simulink model "Modele_LQR_6DOF_EXPERIMENTATION"  (R2024b)
settings: Solver=VariableStepAuto  StartTime=0.0  StopTime=30  FixedStep=0.0001  RelTol=1e-3
values from neighbouring files (symbols this model uses):
  A_num = [0 0 0 0 0 0 0 0 0 0 0 0 ... (144 elements, 12x12)]    [Matrice_A_lineaire.mat]    (also in calcul_matrice_A_lineaire.m = double(A_num); resultats_stabilite.mat; testFinale.m = A_fcn(0, 0, 0, val_rll, val_ptc, val_yw, val_u, val_v, val_w; test_calcalV2.m = double(A_num))
  B = df_dcontrol    [Generate_PyMatrix.m]    (also in Parameters.m = -234.459; instabiliter_graphique.m = out.B_s.signals.values)
  Fx1 = -0.7071*force    (= -0.7071)    [Parameters.m]
  Fx2 = -0.7071*force    (= -0.7071)    [Parameters.m]
  Fx3 = 0    [Parameters.m]
  Fx4 = 0    [Parameters.m]
  Fx5 = 0    [Parameters.m]
  Fx6 = 0    [Parameters.m]
  Fx7 = 0.7071*force    (= 0.7071)    [Parameters.m]
  Fx8 = 0.7071*force    (= 0.7071)    [Parameters.m]
  Fy1 = 0.7071*force    (= 0.7071)    [Parameters.m]
  Fy2 = -0.7071*force    (= -0.7071)    [Parameters.m]
  Fy3 = 0    [Parameters.m]
  Fy4 = 0    [Parameters.m]
  Fy5 = 0    [Parameters.m]
  Fy6 = 0    [Parameters.m]
  Fy7 = 0.7071*force    (= 0.7071)    [Parameters.m]
  Fy8 = -0.7071*force    (= -0.7071)    [Parameters.m]
  Fz1 = 0    [Parameters.m]
  Fz2 = 0    [Parameters.m]
  Fz3 = -1*force    (= -1)    [Parameters.m]
  Fz4 = -1*force    (= -1)    [Parameters.m]
  Fz5 = -1*force    (= -1)    [Parameters.m]
  Fz6 = -1*force    (= -1)    [Parameters.m]
  Fz7 = 0    [Parameters.m]
  Fz8 = 0    [Parameters.m]
  I_x = 0.578    [Parameters.m]
  I_y = 0.645    [Parameters.m]
  I_z = 0.9366    [Parameters.m]
  lx1 = 0.2987    [Parameters.m]
  lx2 = 0.2987    [Parameters.m]
  lx3 = -0.1073    [Parameters.m]
  lx4 = -0.1073    [Parameters.m]
  lx5 = 0.1073    [Parameters.m]
  lx6 = 0.1073    [Parameters.m]
  lx7 = -0.2987    [Parameters.m]
  lx8 = -0.2987    [Parameters.m]
  ly1 = 0.2130    (= 0.213)    [Parameters.m]
  ly2 = -0.2130    (= -0.213)    [Parameters.m]
  ly3 = 0.2725    [Parameters.m]
  ly4 = -0.2725    [Parameters.m]
  ly5 = 0.2725    [Parameters.m]
  ly6 = -0.2725    [Parameters.m]
  ly7 = 0.2130    (= 0.213)    [Parameters.m]
  ly8 = -0.2130    (= -0.213)    [Parameters.m]
  lz1 = 0    [Parameters.m]
  lz2 = 0    [Parameters.m]
  lz3 = 0    [Parameters.m]
  lz4 = 0    [Parameters.m]
  lz5 = 0    [Parameters.m]
  lz6 = 0    [Parameters.m]
  lz7 = 0    [Parameters.m]
  lz8 = 0    [Parameters.m]
  m = 0.427    [Calcul_Inertie_Nouveau.m]    (also in Parameters.m = 23.9)
  Q_envoyer = Q_final(:,:,1)    [Parameters.m]
  W = mass*gravity    (= 234.459)    [Generate_PyMatrix.m]    (also in Parameters.m; calcul_damping.m)
  x_rb = 0    [Parameters.m]
  x_rg = 0    [Parameters.m]
  y_rb = 0    [Parameters.m]
  y_rg = 0    [Parameters.m]
  z_rb = 0    [Parameters.m]
  z_rg = 0    [Parameters.m]
undefined symbols (not defined in the file or in its folder): sigbuilder_block
libraries: simulink x12, sharedtransform x1, dspinverses x1, SignalEditorBlockLib x1
(part 2 of 3)

== matlab function Modele_LQR_6DOF_EXPERIMENTATION/ROV model/ROV model/Kinetics1 ==
  data: u input size=1; u_dot output; v input size=1; w input size=1; p input size=1; q input size=1; r input size=1; phi input; theta input; psi input; tau input; v_dot output; w_dot output; p_dot output; q_dot output; r_dot output; u_dot_temp input; v_dot_temp input; w_dot_temp input; p_dot_temp input; q_dot_temp input; r_dot_temp input; disturbance input; EstimatedParams input; B parameter; Fx1 input; Fx2 input; Fx3 input; Fx4 input; Fx5 input; Fx6 input; Fx7 input; Fx8 input; Fy1 input; Fy2 input; Fy3 input; Fy4 input; Fy5 input; Fy6 input; Fy7 input; Fy8 input; Fz1 input; Fz2 input; Fz3 input; Fz4 input; Fz5 input; Fz6 input; Fz7 input; Fz8 input; I_x input; I_y input; I_z input; lx1 input; lx2 input; lx3 input; lx4 input; lx5 input; lx6 input; lx7 input; lx8 input; ly1 input; ly2 input; ly3 input; ly4 input; ly5 input; ly6 input; ly7 input; ly8 input; lz1 input; lz2 input; lz3 input; lz4 input; lz5 input; lz6 input; lz7 input; lz8 input; m parameter; W parameter; x_rb parameter; x_rg parameter; y_rb parameter; y_rg parameter; z_rb parameter; z_rg parameter; data output; ForceTotal output
function [u_dot, v_dot, w_dot, p_dot, q_dot, r_dot, data, ForceTotal] = Kinetics1( ...
    u, v, w, p, q, r, phi, theta, psi, tau, ...
    u_dot_temp, v_dot_temp, w_dot_temp, p_dot_temp, q_dot_temp, r_dot_temp, ...
    disturbance, EstimatedParams, B, ...
    Fx1, Fx2, Fx3, Fx4, Fx5, Fx6, Fx7, Fx8, ...
    Fy1, Fy2, Fy3, Fy4, Fy5, Fy6, Fy7, Fy8, ...
    Fz1, Fz2, Fz3, Fz4, Fz5, Fz6, Fz7, Fz8, ...
    I_x, I_y, I_z, ...
    lx1, lx2, lx3, lx4, lx5, lx6, lx7, lx8, ...
    ly1, ly2, ly3, ly4, ly5, ly6, ly7, ly8, ...
    lz1, lz2, lz3, lz4, lz5, lz6, lz7, lz8, ...
    m, W, x_rb, x_rg, y_rb, y_rg, z_rb, z_rg)
% ROV 6-DOF Kinetics — Newton-Euler equations (Fossen, p.58)
%
% INPUTS:
%   [u,v,w]         — linear velocities, body frame (m/s)
%   [p,q,r]         — angular velocities, body frame (rad/s)
%   [phi,theta,psi] — Euler angles (rad)
%   tau             — thruster forces (8x1, N)
%   [*_dot_temp]    — previous-step accelerations (breaks angular/linear circularity)
%   disturbance     — current disturbances [uc,vc,wc,pc,qc,rc]
%   EstimatedParams — hydrodynamic coefficients (18x1)
%   B, W            — buoyancy and weight (N)
%   Fx/Fy/Fzi       — unit force direction cosines for thruster i
%   I_x/y/z         — moments of inertia (kg.m²)
%   lx/ly/lzi       — moment arms for thruster i (m)
%   m               — mass (kg)
%   x/y/z_rb/rg     — buoyancy / gravity centre offsets (m)

% ── Constants (hardcoded — remove overrides to use argument values) ───
m    = 23.9;
B    = W;       % neutral buoyancy: (B-W)=0, all gX/gY/gZ terms vanish

x_rg = 0; y_rg = 0; z_rg = 0;
x_rb = 0; y_rb = 0; z_rb = 0;

% ── Previous-step accelerations (avoid circular dependency) ───────────
% p_dot/q_dot/r_dot depend on u_dot/v_dot/w_dot of the same step,
% so we use the delayed integrator feedback values instead.
ud = u_dot_temp;
vd = v_dot_temp;
wd = w_dot_temp;

% ── Hydrodynamic coefficients ─────────────────────────────────────────
X_u  = EstimatedParams(1);   Y_v  = EstimatedParams(2);
Z_w  = EstimatedParams(3);   K_p  = EstimatedParams(4);
M_q  = EstimatedParams(5);   N_r  = EstimatedParams(6);
X_uu = EstimatedParams(7);   Y_vv = EstimatedParams(8);
Z_ww = EstimatedParams(9);   K_pp = EstimatedParams(10);
M_qq = EstimatedParams(11);  N_rr = EstimatedParams(12);
X_ud = EstimatedParams(13);  Y_vd = EstimatedParams(14);
Z_wd = EstimatedParams(15);  K_pd = EstimatedParams(16);
M_qd = EstimatedParams(17);  N_rd = EstimatedParams(18);

% ── Current disturbances ──────────────────────────────────────────────
u_c = disturbance(1);  v_c = disturbance(2);  w_c = disturbance(3);
p_c = disturbance(4);  q_c = disturbance(5);  r_c = disturbance(6);

% ── Relative velocities ───────────────────────────────────────────────
ur = u - u_c;  vr = v - v_c;  wr = w - w_c;
pr = p - p_c;  qr = q - q_c;  rr = r - r_c;

% ── Trig ──────────────────────────────────────────────────────────────
sphi = sin(phi);  cphi = cos(phi);
sth  = sin(theta); cth = cos(theta);

% ── Thruster arrays ───────────────────────────────────────────────────
Fx = [Fx1 Fx2 Fx3 Fx4 Fx5 Fx6 Fx7 Fx8];
Fy = [Fy1 Fy2 Fy3 Fy4 Fy5 Fy6 Fy7 Fy8];
Fz = [Fz1 Fz2 Fz3 Fz4 Fz5 Fz6 Fz7 Fz8];
lx = [lx1 lx2 lx3 lx4 lx5 lx6 lx7 lx8];
ly = [ly1 ly2 ly3 ly4 ly5 ly6 ly7 ly8];
lz = [lz1 lz2 lz3 lz4 lz5 lz6 lz7 lz8];
f  = tau(1:8)';

% ── Generalised thruster forces and moments ───────────────────────────
tauX = sum(Fx .* f);
tauY = sum(Fy .* f);
tauZ = sum(Fz .* f);
tauK = sum((Fy.*lz - Fz.*ly) .* f);
tauM = sum((Fx.*lz - Fz.*lx) .* f);
tauN = sum((Fx.*ly - Fy.*lx) .* f);

% ══════════════════════════════════════════════════════════════════════
% Equations of motion — each variable isolated on the LHS
% All terms reproduced faithfully from original; only layout changed.
% ══════════════════════════════════════════════════════════════════════

% ── u_dot (surge) ────────────────────────────────────────────────────
u_dot = -(  (X_u + X_uu*abs(ur))*ur ...           % damping
          + tauX ...                               % thrusters
          + (q*w_c - r*v_c)*(X_ud - m) ...        % current-rate Coriolis
          + (Z_wd*wr + m*x_rg*qr)*qr ...
          - (Y_vd*vr - m*x_rg*rr)*rr ...
          + sth*(B - W) ...                        % restoring (=0 if B=W)
          - (m*y_rg*qr + m*z_rg*rr)*pr ...
          - m*qr*wr + m*rr*vr ...
          - m*q_dot_temp*z_rg + m*r_dot_temp*y_rg ...
         ) / (X_ud - m);

% ── v_dot (sway) ─────────────────────────────────────────────────────
v_dot = -(  (Y_v + Y_vv*abs(vr))*vr ...
          + tauY ...
          - (p*w_c - r*u_c)*(Y_vd - m) ...
          + (X_ud*ur + m*y_rg*rr)*rr ...
          - (Z_wd*wr - m*y_rg*pr)*pr ...
          - (m*x_rg*pr + m*z_rg*rr)*qr ...
          + m*pr*wr - m*rr*ur ...
          - cth*sphi*(B - W) ...
          + m*p_dot_temp*z_rg - m*r_dot_temp*x_rg ...
         ) / (Y_vd - m);

% ── w_dot (heave) ────────────────────────────────────────────────────
w_dot = -(  (Z_w + Z_ww*abs(wr))*wr ...
          + tauZ ...
          + (p*v_c - q*u_c)*(Z_wd - m) ...
          + (Y_vd*vr + m*z_rg*pr)*pr ...
          - (X_ud*ur - m*z_rg*qr)*qr ...
          - (m*x_rg*pr + m*y_rg*qr)*rr ...
          - m*pr*vr + m*qr*ur ...
          - cphi*cth*(B - W) ...
          - m*p_dot_temp*y_rg + m*q_dot_temp*x_rg ...
         ) / (Z_wd - m);

% ── p_dot (roll) ─────────────────────────────────────────────────────
p_dot = -(  (K_p + K_pp*abs(pr))*pr ...
          + tauK ...
          + (Y_vd*vr + m*z_rg*pr)*wr ...
          - (Z_wd*wr - m*y_rg*pr)*vr ...
          - cth*(W*y_rg*cphi - W*z_rg*sphi - B*y_rb*cphi + B*z_rb*sphi) ...
          - (m*y_rg*qr + m*z_rg*rr)*ur ...
          - (I_y*qr - M_qd*qr)*rr ...
          + (I_z*rr - N_rd*rr)*qr ...
          + m*y_rg*(wd + p*v_c - q*u_c) ...
          - m*z_rg*(vd - p*w_c + r*u_c) ...
         ) / (I_x - K_pd);

% ── q_dot (pitch) ────────────────────────────────────────────────────
q_dot = (   (M_q + M_qq*abs(qr))*qr ...
          + tauM ...
          - (Z_wd*wr + m*x_rg*qr)*ur ...
          + (X_ud*ur - m*z_rg*qr)*wr ...
          - (I_x*pr - K_pd*pr)*rr ...
          + (m*x_rg*pr + m*z_rg*rr)*vr ...
          + (I_z*rr - N_rd*rr)*pr ...
          + B*z_rb*sth - W*z_rg*sth ...
          + m*x_rg*(wd + p*v_c - q*u_c) ...
          - m*z_rg*(ud + q*w_c - r*v_c) ...
          + B*x_rb*cphi*cth - W*x_rg*cphi*cth ...
        ) / (I_y - M_qd);

% ── r_dot (yaw) ──────────────────────────────────────────────────────
r_dot = -(  (N_r + N_rr*abs(rr))*rr ...
          + tauN ...
          + (X_ud*ur + m*y_rg*rr)*vr ...
          - (Y_vd*vr - m*x_rg*rr)*ur ...
          - (I_x*pr - K_pd*pr)*qr ...
          + (I_y*qr - M_qd*qr)*pr ...
          - (m*x_rg*pr + m*y_rg*qr)*wr ...
          + B*y_rb*sth - W*y_rg*sth ...
          + m*x_rg*(vd - p*w_c + r*u_c) ...
          - m*y_rg*(ud + q*w_c - r*v_c) ...
          + B*x_rb*cth*sphi - W*x_rg*cth*sphi ...
         ) / (I_z - N_rd);

data = [ ...
u v w p q r ...
ur vr wr pr qr rr ...
u_dot v_dot w_dot p_dot q_dot r_dot];
ForceTotal = [tauX tauY tauZ tauK tauM tauN];
end

== matlab function Modele_LQR_6DOF_EXPERIMENTATION/Controller/MATLAB Function ==
  settings: updateMethod=DISCRETE
  data: R output; Q output; A output; B output; state input; Q_files input; A_lineraire input

function [R,Q,A,B]= ABmatrix(state, Q_files, A_lineraire)
tic
    
    roll_ = state(4);
    pitch_ = state(5);
    yaw_ = state(6);
    u = state(7); %
    v = state(8); %
    w = state(9); %
    p = state(10);
    q = state(11);
    r = state(12);
    thrust = 10;
    importance = 0;

    % Q = Q_files;
    Q = diag([Q_files(1,1)+200 Q_files(2,2)+200 Q_files(3,3)+200 Q_files(4,4) Q_files(5,5) Q_files(6,6) Q_files(7,7) Q_files(8,8) Q_files(9,9) Q_files(10,10) Q_files(11,11) Q_files(12,12)]);
    % Q = diag([80, 80, 80, 40, 40, 40, 20, 20, 20, 20, 20, 20]); % test répétition
    % Q = diag([4, 4, 4, 2, 2, 2, 1, 1, 1, 1, 1, 1]); % test ancien
    % R = diag([thrust, thrust, thrust-importance, thrust-importance, thrust-importance, thrust-importance, thrust, thrust]); 
    R = thrust*eye(8);

    radius = 0.26;
    
 % A = A_lineraire;

 % utiliser
%     A = [[0, 0, 0,   v*(sin(roll_)*sin(yaw_) + cos(roll_)*cos(yaw_)*sin(pitch_)) + w*(cos(roll_)*sin(yaw_) - cos(yaw_)*sin(pitch_)*sin(roll_)), w*cos(pitch_)*cos(roll_)*cos(yaw_) - u*cos(yaw_)*sin(pitch_) + v*cos(pitch_)*cos(yaw_)*sin(roll_), w*(cos(yaw_)*sin(roll_) - cos(roll_)*sin(pitch_)*sin(yaw_)) - v*(cos(roll_)*cos(yaw_) + sin(pitch_)*sin(roll_)*sin(yaw_)) - u*cos(pitch_)*sin(yaw_), cos(pitch_)*cos(yaw_), cos(yaw_)*sin(pitch_)*sin(roll_) - cos(roll_)*sin(yaw_), sin(roll_)*sin(yaw_) + cos(roll_)*cos(yaw_)*sin(pitch_),             0,                      0,                      0]
% [0, 0, 0, - v*(cos(yaw_)*sin(roll_) - cos(roll_)*sin(pitch_)*sin(yaw_)) - w*(cos(roll_)*cos(yaw_) + sin(pitch_)*sin(roll_)*sin(yaw_)), w*cos(pitch_)*cos(roll_)*sin(yaw_) - u*sin(pitch_)*sin(yaw_) + v*cos(pitch_)*sin(roll_)*sin(yaw_), w*(sin(roll_)*sin(yaw_) + cos(roll_)*cos(yaw_)*sin(pitch_)) - v*(cos(roll_)*sin(yaw_) - cos(yaw_)*sin(pitch_)*sin(roll_)) + u*cos(pitch_)*cos(yaw_), cos(pitch_)*sin(yaw_), cos(roll_)*cos(yaw_) + sin(pitch_)*sin(roll_)*sin(yaw_), cos(roll_)*sin(pitch_)*sin(yaw_) - cos(yaw_)*sin(roll_),             0,                      0,                      0]
% [0, 0, 0,                                                                         v*cos(pitch_)*cos(roll_) - w*cos(pitch_)*sin(roll_),                             - u*cos(pitch_) - w*cos(roll_)*sin(pitch_) - v*sin(pitch_)*sin(roll_),                                                                                                                                                   0,          -sin(pitch_),                                  cos(pitch_)*sin(roll_),                                  cos(pitch_)*cos(roll_),             0,                      0,                      0]
% [0, 0, 0,                                                                         q*cos(roll_)*tan(pitch_) - r*tan(pitch_)*sin(roll_),                               r*cos(roll_)*(tan(pitch_)^2 + 1) + q*sin(roll_)*(tan(pitch_)^2 + 1),                                                                                                                                                   0,                     0,                                                       0,                                                       0,             1, tan(pitch_)*sin(roll_), cos(roll_)*tan(pitch_)]
% [0, 0, 0,                                                                                               - r*cos(roll_) - q*sin(roll_),                                                                                                 0,                                                                                                                                                   0,                     0,                                                       0,                                                       0,             0,             cos(roll_),            -sin(roll_)]
% [0, 0, 0,                                                                     (q*cos(roll_))/cos(pitch_) - (r*sin(roll_))/cos(pitch_),               (r*cos(roll_)*sin(pitch_))/cos(pitch_)^2 + (q*sin(pitch_)*sin(roll_))/cos(pitch_)^2,                                                                                                                                                   0,                     0,                                                       0,                                                       0,             0, sin(roll_)/cos(pitch_), cos(roll_)/cos(pitch_)]
% [0, 0, 0,                                                                                                                           0,                                            (10*cos(pitch_)*(13080*pi*radius^3 - 234459/1000))/139,                                                                                                                                                   0,            -2221/1390,                                                       r,                                                      -q,             0,                     -w,                      v]
% [0, 0, 0,                                                          -(10*cos(pitch_)*cos(roll_)*(13080*pi*radius^3 - 234459/1000))/139,                                 (10*sin(pitch_)*sin(roll_)*(13080*pi*radius^3 - 234459/1000))/139,                                                                                                                                                   0,                    -r,                                               -1394/695,                                                       p,             w,                      0,                     -u]
% [0, 0, 0,                                                           (10*cos(pitch_)*sin(roll_)*(13080*pi*radius^3 - 234459/1000))/139,                                 (10*cos(roll_)*sin(pitch_)*(13080*pi*radius^3 - 234459/1000))/139,                                                                                                                                                   0,                     q,                                                      -p,                                               -2107/695,            -v,                      u,                      0]
% [0, 0, 0,                                                                                                                           0,                                                                                                 0,                                                                                                                                                   0,                     0,                                                       0,                                                       0, -193590/40171,           -(146*r)/289,           -(146*q)/289]
% [0, 0, 0,                                                                                                                           0,                                                                                                 0,                                                                                                                                                   0,                     0,                                                       0,                                                       0,   (359*r)/645,            -25812/5977,            (359*p)/645]
% [0, 0, 0,                                                                                                                           0,                                                                                                 0,                                                                                                                                                   0,                     0,                                                       0,                                                       0,   -(67*q)/937,            -(67*p)/937,         -387180/130243]];

% A displace wather 0.0147

    A = [[0, 0, 0,   v*(sin(roll_)*sin(yaw_) + cos(roll_)*cos(yaw_)*sin(pitch_)) + w*(cos(roll_)*sin(yaw_) - cos(yaw_)*sin(pitch_)*sin(roll_)), w*cos(pitch_)*cos(roll_)*cos(yaw_) - u*cos(yaw_)*sin(pitch_) + v*cos(pitch_)*cos(yaw_)*sin(roll_), w*(cos(yaw_)*sin(roll_) - cos(roll_)*sin(pitch_)*sin(yaw_)) - v*(cos(roll_)*cos(yaw_) + sin(pitch_)*sin(roll_)*sin(yaw_)) - u*cos(pitch_)*sin(yaw_), cos(pitch_)*cos(yaw_), cos(yaw_)*sin(pitch_)*sin(roll_) - cos(roll_)*sin(yaw_), sin(roll_)*sin(yaw_) + cos(roll_)*cos(yaw_)*sin(pitch_),                                             0,                                              0,                                              0]
[0, 0, 0, - v*(cos(yaw_)*sin(roll_) - cos(roll_)*sin(pitch_)*sin(yaw_)) - w*(cos(roll_)*cos(yaw_) + sin(pitch_)*sin(roll_)*sin(yaw_)), w*cos(pitch_)*cos(roll_)*sin(yaw_) - u*sin(pitch_)*sin(yaw_) + v*cos(pitch_)*sin(roll_)*sin(yaw_), w*(sin(roll_)*sin(yaw_) + cos(roll_)*cos(yaw_)*sin(pitch_)) - v*(cos(roll_)*sin(yaw_) - cos(yaw_)*sin(pitch_)*sin(roll_)) + u*cos(pitch_)*cos(yaw_), cos(pitch_)*sin(yaw_), cos(roll_)*cos(yaw_) + sin(pitch_)*sin(roll_)*sin(yaw_), cos(roll_)*sin(pitch_)*sin(yaw_) - cos(yaw_)*sin(roll_),                                             0,                                              0,                                              0]
[0, 0, 0,                                                                         v*cos(pitch_)*cos(roll_) - w*cos(pitch_)*sin(roll_),                             - u*cos(pitch_) - w*cos(roll_)*sin(pitch_) - v*sin(pitch_)*sin(roll_),                                                                                                                                                   0,          -sin(pitch_),                                  cos(pitch_)*sin(roll_),                                  cos(pitch_)*cos(roll_),                                             0,                                              0,                                              0]
[0, 0, 0,                                                                         q*cos(roll_)*tan(pitch_) - r*tan(pitch_)*sin(roll_),                               r*cos(roll_)*(tan(pitch_)^2 + 1) + q*sin(roll_)*(tan(pitch_)^2 + 1),                                                                                                                                                   0,                     0,                                                       0,                                                       0,                                             1,                         tan(pitch_)*sin(roll_),                         cos(roll_)*tan(pitch_)]
[0, 0, 0,                                                                                               - r*cos(roll_) - q*sin(roll_),                                                                                                 0,                                                                                                                                                   0,                     0,                                                       0,                                                       0,                                             0,                                     cos(roll_),                                    -sin(roll_)]
[0, 0, 0,                                                                     (q*cos(roll_))/cos(pitch_) - (r*sin(roll_))/cos(pitch_),               (r*cos(roll_)*sin(pitch_))/cos(pitch_)^2 + (q*sin(pitch_)*sin(roll_))/cos(pitch_)^2,                                                                                                                                                   0,                     0,                                                       0,                                                       0,                                             0,                         sin(roll_)/cos(pitch_),                         cos(roll_)/cos(pitch_)]
[0, 0, 0,                                                                                                                           0,                                              (5*cos(pitch_)*(13080*pi*radius^3 - 234459/1000))/46,                                                                                                                                                   0,             -2221/920,                                                       r,                                                      -q,                                             0,                                             -w,                                              v]
[0, 0, 0,                                                            -(5*cos(pitch_)*cos(roll_)*(13080*pi*radius^3 - 234459/1000))/46,                                   (5*sin(pitch_)*sin(roll_)*(13080*pi*radius^3 - 234459/1000))/46,                                                                                                                                                   0,                    -r,                                                -697/230,                                                       p,                                             w,                                              0,                                             -u]
[0, 0, 0,                                                             (5*cos(pitch_)*sin(roll_)*(13080*pi*radius^3 - 234459/1000))/46,                                   (5*cos(roll_)*sin(pitch_)*(13080*pi*radius^3 - 234459/1000))/46,                                                                                                                                                   0,                     q,                                                      -p,                                               -2107/460,                                            -v,                                              u,                                              0]
[0, 0, 0,                                                                                                                           0,                                                                                                 0,                                                                                                                                                   0,                     0,                                                       0,                                                       0,        -911978924542525440/125252831477538461, -(15123087548710128886*r)/29935426723131692179, -(15123087548710128886*q)/29935426723131692179]
[0, 0, 0,                                                                                                                           0,                                                                                                 0,                                                                                                                                                   0,                     0,                                                       0,                                                       0,  (6197703687199696929*r)/11135150078673551360,                                      -6453/989,   (6197703687199696929*p)/11135150078673551360]
[0, 0, 0,                                                                                                                           0,                                                                                                 0,                                                                                                                                                   0,                     0,                                                       0,                                                       0, -(3470023512888961901*q)/48528537784730782966,  -(3470023512888961901*p)/48528537784730782966,         -455989462271262720/101524137624959797]];

% original
%     A = [[ 0, 0, 0,   v*(sin(roll_)*sin(yaw_) + cos(roll_)*cos(yaw_)*sin(pitch_)) + w*(cos(roll_)*sin(yaw_) - cos(yaw_)*sin(pitch_)*sin(roll_)), w*cos(pitch_)*cos(roll_)*cos(yaw_) - u*cos(yaw_)*sin(pitch_) + v*cos(pitch_)*cos(yaw_)*sin(roll_), w*(cos(yaw_)*sin(roll_) - cos(roll_)*sin(pitch_)*sin(yaw_)) - v*(cos(roll_)*cos(yaw_) + sin(pitch_)*sin(roll_)*sin(yaw_)) - u*cos(pitch_)*sin(yaw_), cos(pitch_)*cos(yaw_), cos(yaw_)*sin(pitch_)*sin(roll_) - cos(roll_)*sin(yaw_), sin(roll_)*sin(yaw_) + cos(roll_)*cos(yaw_)*sin(pitch_),          0,                      0,                      0]
% [ 0, 0, 0, - v*(cos(yaw_)*sin(roll_) - cos(roll_)*sin(pitch_)*sin(yaw_)) - w*(cos(roll_)*cos(yaw_) + sin(pitch_)*sin(roll_)*sin(yaw_)), w*cos(pitch_)*cos(roll_)*sin(yaw_) - u*sin(pitch_)*sin(yaw_) + v*cos(pitch_)*sin(roll_)*sin(yaw_), w*(sin(roll_)*sin(yaw_) + cos(roll_)*cos(yaw_)*sin(pitch_)) - v*(cos(roll_)*sin(yaw_) - cos(yaw_)*sin(pitch_)*sin(roll_)) + u*cos(pitch_)*cos(yaw_), cos(pitch_)*sin(yaw_), cos(roll_)*cos(yaw_) + sin(pitch_)*sin(roll_)*sin(yaw_), cos(roll_)*sin(pitch_)*sin(yaw_) - cos(yaw_)*sin(roll_),          0,                      0,                      0]
% [ 0, 0, 0,                                                                         v*cos(pitch_)*cos(roll_) - w*cos(pitch_)*sin(roll_),                             - u*cos(pitch_) - w*cos(roll_)*sin(pitch_) - v*sin(pitch_)*sin(roll_),                                                                                                                                                   0,          -sin(pitch_),                                  cos(pitch_)*sin(roll_),                                  cos(pitch_)*cos(roll_),          0,                      0,                      0]
% [ 0, 0, 0,                                                                         q*cos(roll_)*tan(pitch_) - r*tan(pitch_)*sin(roll_),                               r*cos(roll_)*(tan(pitch_)^2 + 1) + q*sin(roll_)*(tan(pitch_)^2 + 1),                                                                                                                                                   0,                     0,                                                       0,                                                       0,          1, tan(pitch_)*sin(roll_), cos(roll_)*tan(pitch_)]
% [ 0, 0, 0,                                                                                               - r*cos(roll_) - q*sin(roll_),                                                                                                 0,                                                                                                                                                   0,                     0,                                                       0,                                                       0,          0,             cos(roll_),            -sin(roll_)]
% [ 0, 0, 0,                                                                     (q*cos(roll_))/cos(pitch_) - (r*sin(roll_))/cos(pitch_),               (r*cos(roll_)*sin(pitch_))/cos(pitch_)^2 + (q*sin(pitch_)*sin(roll_))/cos(pitch_)^2,                                                                                                                                                   0,                     0,                                                       0,                                                       0,          0, sin(roll_)/cos(pitch_), cos(roll_)/cos(pitch_)]
% [ 0, 0, 0,                                                                                                                           0,                                                    (7873445366256113*cos(pitch_))/395824185999360,                                                                                                                                                   0,             2221/2250,                                               (17*r)/25,                                          -(1343*q)/2250,          0,         -(1343*w)/2250,              (17*v)/25]
% [ 0, 0, 0,                                                                   -(2315719225369445*cos(pitch_)*cos(roll_))/79164837199872,                                          (2315719225369445*sin(pitch_)*sin(roll_))/79164837199872,                                                                                                                                                   0,            -(25*r)/17,                                                   82/45,                                               (79*p)/90,  (79*w)/90,                      0,             -(25*u)/17]
% [ 0, 0, 0,                                                                      (146564507934775*cos(pitch_)*sin(roll_))/4398046511104,                                            (146564507934775*cos(roll_)*sin(pitch_))/4398046511104,                                                                                                                                                   0,         (2250*q)/1343,                                              -(90*p)/79,                                               4214/1343, -(90*v)/79,          (2250*u)/1343,                      0]
% [ 0, 0, 0,                                                                                                                           0,                                                                                                 0,                                                                                                                                                   0,                     0,                                               (187*w)/4,                                               (187*v)/4,       81/2,                      0,                      0]
% [ 0, 0, 0,                                                                                                                           0,                                                                                                 0,                                                                                                                                                   0,            -(907*w)/4,                                                       0,                                              -(907*u)/4,          0,                   81/2,                      0]
% [ 0, 0, 0,                                                                                                                           0,                                                                                                 0,                                                                                                                                                   0,                 180*v,                                                   180*u,                                                       0,          0,                      0,                   81/2]];

% utiliser
%     B = [[                                          0,                                            0,              0,              0,             0,             0,                                            0,                                           0]
% [                                          0,                                            0,              0,              0,             0,             0,                                            0,                                           0]
% [                                          0,                                            0,              0,              0,             0,             0,                                            0,                                           0]
% [                                          0,                                            0,              0,              0,             0,             0,                                            0,                                           0]
% [                                          0,                                            0,              0,              0,             0,             0,                                            0,                                           0]
% [                                          0,                                            0,              0,              0,             0,             0,                                            0,                                           0]
% [                                  -707/6950,                                    -707/6950,              0,              0,             0,             0,                                     707/6950,                                    707/6950]
% [                                   707/6950,                                    -707/6950,              0,              0,             0,             0,                                     707/6950,                                   -707/6950]
% [                                          0,                                            0,        -20/139,        -20/139,       -20/139,       -20/139,                                            0,                                           0]
% [                                          0,                                            0,  -130255/80342,   130255/80342, -130255/80342,  130255/80342,                                            0,                                           0]
% [                                          0,                                            0, -256447/448275, -256447/448275, 256447/448275, 256447/448275,                                            0,                                           0]
% [194698457386957391875/146640581566903877632, -194698457386957391875/146640581566903877632,              0,              0,             0,             0, -194698457386957391875/146640581566903877632, 194698457386957391875/146640581566903877632]];

% matrice B displace wather 0.0147

    B = [[                                    0,                                      0,                                      0,                                     0,                                      0,                                     0,                                      0,                                     0]
[                                    0,                                      0,                                      0,                                     0,                                      0,                                     0,                                      0,                                     0]
[                                    0,                                      0,                                      0,                                     0,                                      0,                                     0,                                      0,                                     0]
[                                    0,                                      0,                                      0,                                     0,                                      0,                                     0,                                      0,                                     0]
[                                    0,                                      0,                                      0,                                     0,                                      0,                                     0,                                      0,                                     0]
[                                    0,                                      0,                                      0,                                     0,                                      0,                                     0,                                      0,                                     0]
[                            -707/4600,                              -707/4600,                                      0,                                     0,                                      0,                                     0,                               707/4600,                              707/4600]
[                             707/4600,                              -707/4600,                                      0,                                     0,                                      0,                                     0,                               707/4600,                             -707/4600]
[                                    0,                                      0,                                  -5/23,                                 -5/23,                                  -5/23,                                 -5/23,                                      0,                                     0]
[                                    0,                                      0, -306807724614615040/125252831477538461, 306807724614615040/125252831477538461, -306807724614615040/125252831477538461, 306807724614615040/125252831477538461,                                      0,                                     0]
[                                    0,                                      0,                         -256447/296700,                        -256447/296700,                          256447/296700,                         256447/296700,                                      0,                                     0]
[814637897016558125/406096550499839188, -814637897016558125/406096550499839188,                                      0,                                     0,                                      0,                                     0, -814637897016558125/406096550499839188, 814637897016558125/406096550499839188]]; 


% matrice original
%     B = [[                                   0,                                    0,         0,         0,         0,         0,                                    0,                                   0]
% [                                   0,                                    0,         0,         0,         0,         0,                                    0,                                   0]
% [                                   0,                                    0,         0,         0,         0,         0,                                    0,                                   0]
% [                                   0,                                    0,         0,         0,         0,         0,                                    0,                                   0]
% [                                   0,                                    0,         0,         0,         0,         0,                                    0,                                   0]
% [                                   0,                                    0,         0,         0,         0,         0,                                    0,                                   0]
% [                          -707/11250,                           -707/11250,         0,         0,         0,         0,                            707/11250,                           707/11250]
% [                            707/7650,                            -707/7650,         0,         0,         0,         0,                             707/7650,                           -707/7650]
% [                                   0,                                    0, -200/1343, -200/1343, -200/1343, -200/1343,                                    0,                                   0]
% [                                   0,                                    0,    -109/8,     109/8,    -109/8,     109/8,                                    0,                                   0]
% [                                   0,                                    0, -1073/200, -1073/200,  1073/200,  1073/200,                                    0,                                   0]
% [ 162927579403311625/9007199254740992, -162927579403311625/9007199254740992,         0,         0,         0,         0, -162927579403311625/9007199254740992, 162927579403311625/9007199254740992]];

toc
end

== matlab function Modele_LQR_6DOF_EXPERIMENTATION/Thrustherforces in newtons/MATLAB Function1 ==
  data: u input; tau output
function tau = fcn(u)
%#codegen
lookup =[...
    -40.0337   -1.0000
    -40.0337   -0.9750
    -40.0788   -0.9500
    -37.5428   -0.9250
    -36.6092   -0.9000
    -35.4971   -0.8750
    -33.7623   -0.8500
    -32.3835   -0.8250
    -31.2263   -0.8000
    -29.9809   -0.7750
    -28.5128   -0.7500
    -27.6234   -0.7250
    -26.5554   -0.7000
    -24.7765   -0.6750
    -23.1751   -0.6500
    -22.1522   -0.6250
    -21.3510   -0.6000
    -19.5280   -0.5750
    -18.4600   -0.5500
    -17.3480   -0.5250
    -16.1025   -0.5000
    -14.6345   -0.4750
    -13.0781   -0.4500
    -12.1877   -0.4250
    -10.9874   -0.4000
    -10.0528   -0.3750
    -8.8966   -0.3500
    -7.7404   -0.3250
    -6.8058   -0.3000
    -6.0497   -0.2750
    -5.1151   -0.2500
    -4.2698   -0.2250
    -3.4696   -0.2000
    -2.7135   -0.1750
    -1.8682   -0.1500
    -1.1121   -0.1250
    -0.5335   -0.1000
    -0.2667   -0.0750
    0   -0.0500
    0   -0.0250
    0         0
    0    0.0250
    0    0.0500
    0.5786    0.0750
    1.1121    0.1000
    1.8240    0.1250
    2.5801    0.1500
    3.4255    0.1750
    4.0923    0.2000
    5.1151    0.2250
    6.2272    0.2500
    7.0284    0.2750
    8.2739    0.3000
    9.2526    0.3250
    10.8089    0.3500
    12.2328    0.3750
    13.6558    0.4000
    14.9904    0.4250
    16.4585    0.4500
    17.7039    0.4750
    19.2161    0.5000
    20.5508    0.5250
    21.7521    0.5500
    23.6644    0.5750
    24.7324    0.6000
    26.4221    0.6250
    27.7126    0.6500
    29.6249    0.6750
    31.3156    0.7000
    32.8729    0.7250
    33.8065    0.7500
    34.2517    0.7750
    37.0534    0.8000
    38.6549    0.8250
    39.2776    0.8500
    41.1458    0.8750
    42.9257    0.9000
    44.7938    0.9250
    47.1062    0.9500
    48.0408    0.9750
    49.9531    1.0000];
%Thrustherforce in newtons.
tau = zeros(8,1);
tau(1) = interp1(lookup(:,2),lookup(:,1),u(1));
tau(2) = interp1(lookup(:,2),lookup(:,1),u(2));
tau(3) = interp1(lookup(:,2),lookup(:,1),u(3));
tau(4) = interp1(lookup(:,2),lookup(:,1),u(4));
tau(5) = interp1(lookup(:,2),lookup(:,1),u(5));
tau(6) = interp1(lookup(:,2),lookup(:,1),u(6));
tau(7) = interp1(lookup(:,2),lookup(:,1),u(7));
tau(8) = interp1(lookup(:,2),lookup(:,1),u(8));

end

== matlab function Modele_LQR_6DOF_EXPERIMENTATION/ROV model/ROV model/Kinematics 2 ==
  data: u_b input; u_n output; v_b input; w_b input; p_b input; q_b input; r_b input; phi input; theta input; psi input; v_n output; w_n output; p_n output; q_n output; r_n output
function [u_n,v_n,w_n,p_n,q_n,r_n] = Kinematics(u_b,v_b,w_b,p_b,q_b,r_b,phi,theta,psi)
% LIVRE HMCH PAGE 27
cphi = cos(phi);
sphi = sin(phi);
cth  = cos(theta);
sth  = sin(theta);
cpsi = cos(psi);
spsi = sin(psi);
tanth = tan(theta);
if cth==0
    error('T is singular for theta = +-90 degrees');
end
 
u_n = u_b*cpsi*cth + v_b*(cpsi*sphi*sth - cphi*spsi) + w_b*(sphi*spsi + cphi*cpsi*sth) ;
v_n = u_b*cth*spsi + v_b*(cphi*cpsi + sphi*spsi*sth) + w_b*(cphi*spsi*sth - cpsi*sphi);
w_n = -u_b*sth+ v_b*cth*sphi + w_b*cphi*cth;
p_n = p_b + q_b*sphi*(tanth) + r_b*cphi*(tanth);
q_n = q_b*cphi - r_b*sphi;
r_n = q_b*(sphi/cth) + r_b*(cphi/cth);


end

== matlab function Modele_LQR_6DOF_EXPERIMENTATION/Controller/LQR/MATLAB Function ==
  settings: updateMethod=DISCRETE
  data: dXdt output; X input; A input; B input; R input; Q input
function dXdt  = mRiccati(X, A, B,R,Q)
% r1=randi([1 1000]);
% r2=randi([1 1000]);
% r3=randi([1 1000]);
% r4=randi([1 1000]);
% r5=randi([1 1000]);
% r6=randi([1 1000]);
% Q = diag([r1 r2 r3 r4 r5 r6] );
% R = 1*diag([1 1 1 1]);
%X = reshape(X, size(A)); %Convert from "n^2"-by-1 to "n"-by-"n"
dXdt = A.'*X + X*A - (X*B)*inv(R)*(B.'*X) + Q; %Determine derivative
% dXdtS= dXdt(:); %Convert from "n"-by-"n" to "n^2"-by-1,algebraic Riccati equation (ARE)

== matlab function Modele_LQR_6DOF_EXPERIMENTATION/MATLAB Function ==
  data: Position input; srf_in input
function Visualize(Position, srf_in)

    coder.extrinsic('setax'); 
    setax(Position, srf_in);  

end

== matlab function Modele_LQR_6DOF_EXPERIMENTATION/Controller/Gestionnaire des Vitesses/MATLAB Function2 ==
  data: xstate input; u output; xtarget input
function u = fcn(xstate,xtarget)

precition = 0.01;
% precition = 0.01; % original

if(xstate < xtarget - precition)
    u = 1; % original (1)

elseif(xstate > xtarget + precition)
    u = -1; % original (-1)
    
else
    u = 0;
end
end

== matlab function Modele_LQR_6DOF_EXPERIMENTATION/Controller/Gestionnaire des Vitesses/MATLAB Function3 ==
  data: xstate input; u output; xtarget input
function u = fcn(xstate,xtarget)

precition = 0.05;
% precition = 0.05; % original

if(xstate < xtarget - precition)
    u = 0.5; % 0.5

elseif(xstate > xtarget + precition)
    u = -0.5;
    
else
    u = 0;
end
end

== matlab function Modele_LQR_6DOF_EXPERIMENTATION/Controller/Gestionnaire des Vitesses/MATLAB Function4 ==
  data: xstate input; u output; xtarget input
function u = fcn(xstate,xtarget)

precition = 0.05;
% precition = 0.05; % original

if(xstate < xtarget - precition)
    u = 0.5; % 0.5

elseif(xstate > xtarget + precition)
    u = -0.5;
    
else
    u = 0;
end
end

== matlab function Modele_LQR_6DOF_EXPERIMENTATION/Controller/Gestionnaire des Vitesses/MATLAB Function5 ==
  data: xstate input; u output; xtarget input
function u = fcn(xstate,xtarget)

precition = 0.02;
% precition = 0.02; % originalt

if(xstate < xtarget - precition)
    u = 0.2; % avant 0.2

elseif(xstate > xtarget + precition)
    u = -0.2;
    
else
    u = 0;
end
end
